simulink library "monroe_library"  (R2012b)
settings: Solver=ode45  StartTime=0.0  StopTime=10.0  RelTol=1e-3
values from neighbouring files (symbols this model uses):
  input_bit_width = ', num2str(input_bit_width))    [fft_direct_draw.m]
undefined symbols (not defined in the file or in its folder): gcbh, xlBlockLoadCallback
libraries: xbsIndex_r4 x1880, monroe_library x159, casper_library x13, xps_library x1
(part 35 of 43)

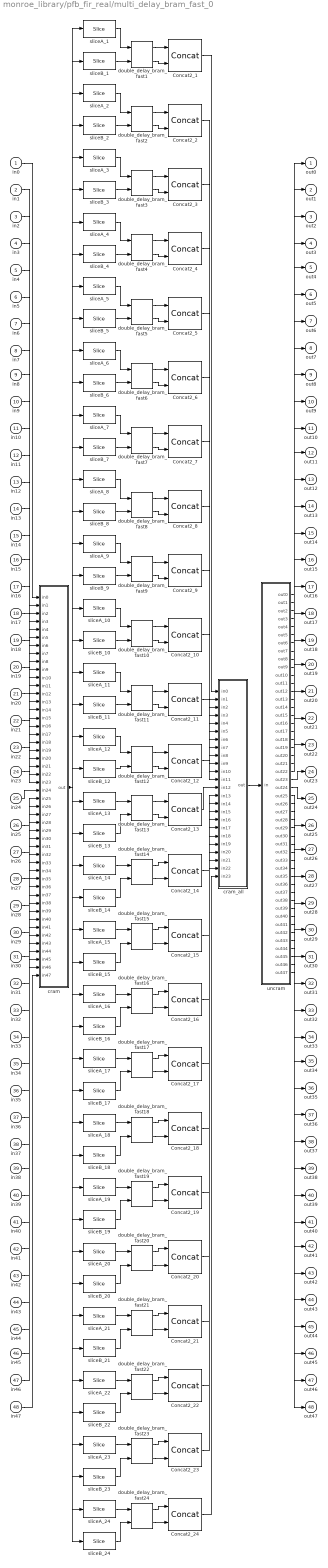
== system monroe_library/pfb_fir_real/multi_delay_bram_fast_0 ==
  in0 : Inport
  in1 : Inport  Port=2
  in2 : Inport  Port=3
  in3 : Inport  Port=4
  in4 : Inport  Port=5
  in5 : Inport  Port=6
  in6 : Inport  Port=7
  in7 : Inport  Port=8
  in8 : Inport  Port=9
  in9 : Inport  Port=10
  in10 : Inport  Port=11
  in11 : Inport  Port=12
  in12 : Inport  Port=13
  in13 : Inport  Port=14
  in14 : Inport  Port=15
  in15 : Inport  Port=16
  in16 : Inport  Port=17
  in17 : Inport  Port=18
  in18 : Inport  Port=19
  in19 : Inport  Port=20
  in20 : Inport  Port=21
  in21 : Inport  Port=22
  in22 : Inport  Port=23
  in23 : Inport  Port=24
  in24 : Inport  Port=25
  in25 : Inport  Port=26
  in26 : Inport  Port=27
  in27 : Inport  Port=28
  in28 : Inport  Port=29
  in29 : Inport  Port=30
  in30 : Inport  Port=31
  in31 : Inport  Port=32
  in32 : Inport  Port=33
  in33 : Inport  Port=34
  in34 : Inport  Port=35
  in35 : Inport  Port=36
  in36 : Inport  Port=37
  in37 : Inport  Port=38
  in38 : Inport  Port=39
  in39 : Inport  Port=40
  in40 : Inport  Port=41
  in41 : Inport  Port=42
  in42 : Inport  Port=43
  in43 : Inport  Port=44
  in44 : Inport  Port=45
  in45 : Inport  Port=46
  in46 : Inport  Port=47
  in47 : Inport  Port=48
  Concat2_{1..24} (24 alike) : xbsIndex_r4/Concat  num_inputs=2  dbl_ovrd=off  block_type=concat
  cram : Subsystem
  cram_all : Subsystem
  double_delay_bram_fast{1..24} (24 alike) : monroe_library/double_delay_bram_fast  SystemSampleTime=-1  delay_len=1024  bram_latency=2  register_counter=0
  sliceA_1 : xbsIndex_r4/Slice  nbits=18  boolean_output=off  mode=Upper Bit Location + Width  bit1=-0  base1=MSB of Input  bit0=-0  base0=MSB of Input  dbl_ovrd=off  block_type=slice
  sliceA_10 : xbsIndex_r4/Slice  nbits=18  boolean_output=off  mode=Upper Bit Location + Width  bit1=-324  base1=MSB of Input  bit0=-324  base0=MSB of Input  dbl_ovrd=off  block_type=slice
  sliceA_11 : xbsIndex_r4/Slice  nbits=18  boolean_output=off  mode=Upper Bit Location + Width  bit1=-360  base1=MSB of Input  bit0=-360  base0=MSB of Input  dbl_ovrd=off  block_type=slice
  sliceA_12 : xbsIndex_r4/Slice  nbits=18  boolean_output=off  mode=Upper Bit Location + Width  bit1=-396  base1=MSB of Input  bit0=-396  base0=MSB of Input  dbl_ovrd=off  block_type=slice
  sliceA_13 : xbsIndex_r4/Slice  nbits=18  boolean_output=off  mode=Upper Bit Location + Width  bit1=-432  base1=MSB of Input  bit0=-432  base0=MSB of Input  dbl_ovrd=off  block_type=slice
  sliceA_14 : xbsIndex_r4/Slice  nbits=18  boolean_output=off  mode=Upper Bit Location + Width  bit1=-468  base1=MSB of Input  bit0=-468  base0=MSB of Input  dbl_ovrd=off  block_type=slice
  sliceA_15 : xbsIndex_r4/Slice  nbits=18  boolean_output=off  mode=Upper Bit Location + Width  bit1=-504  base1=MSB of Input  bit0=-504  base0=MSB of Input  dbl_ovrd=off  block_type=slice
  sliceA_16 : xbsIndex_r4/Slice  nbits=18  boolean_output=off  mode=Upper Bit Location + Width  bit1=-540  base1=MSB of Input  bit0=-540  base0=MSB of Input  dbl_ovrd=off  block_type=slice
  sliceA_17 : xbsIndex_r4/Slice  nbits=18  boolean_output=off  mode=Upper Bit Location + Width  bit1=-576  base1=MSB of Input  bit0=-576  base0=MSB of Input  dbl_ovrd=off  block_type=slice
  sliceA_18 : xbsIndex_r4/Slice  nbits=18  boolean_output=off  mode=Upper Bit Location + Width  bit1=-612  base1=MSB of Input  bit0=-612  base0=MSB of Input  dbl_ovrd=off  block_type=slice
  sliceA_19 : xbsIndex_r4/Slice  nbits=18  boolean_output=off  mode=Upper Bit Location + Width  bit1=-648  base1=MSB of Input  bit0=-648  base0=MSB of Input  dbl_ovrd=off  block_type=slice
  sliceA_2 : xbsIndex_r4/Slice  nbits=18  boolean_output=off  mode=Upper Bit Location + Width  bit1=-36  base1=MSB of Input  bit0=-36  base0=MSB of Input  dbl_ovrd=off  block_type=slice
  sliceA_20 : xbsIndex_r4/Slice  nbits=18  boolean_output=off  mode=Upper Bit Location + Width  bit1=-684  base1=MSB of Input  bit0=-684  base0=MSB of Input  dbl_ovrd=off  block_type=slice
  sliceA_21 : xbsIndex_r4/Slice  nbits=18  boolean_output=off  mode=Upper Bit Location + Width  bit1=-720  base1=MSB of Input  bit0=-720  base0=MSB of Input  dbl_ovrd=off  block_type=slice
  sliceA_22 : xbsIndex_r4/Slice  nbits=18  boolean_output=off  mode=Upper Bit Location + Width  bit1=-756  base1=MSB of Input  bit0=-756  base0=MSB of Input  dbl_ovrd=off  block_type=slice
  sliceA_23 : xbsIndex_r4/Slice  nbits=18  boolean_output=off  mode=Upper Bit Location + Width  bit1=-792  base1=MSB of Input  bit0=-792  base0=MSB of Input  dbl_ovrd=off  block_type=slice
  sliceA_24 : xbsIndex_r4/Slice  nbits=18  boolean_output=off  mode=Upper Bit Location + Width  bit1=-828  base1=MSB of Input  bit0=-828  base0=MSB of Input  dbl_ovrd=off  block_type=slice
  sliceA_3 : xbsIndex_r4/Slice  nbits=18  boolean_output=off  mode=Upper Bit Location + Width  bit1=-72  base1=MSB of Input  bit0=-72  base0=MSB of Input  dbl_ovrd=off  block_type=slice
  sliceA_4 : xbsIndex_r4/Slice  nbits=18  boolean_output=off  mode=Upper Bit Location + Width  bit1=-108  base1=MSB of Input  bit0=-108  base0=MSB of Input  dbl_ovrd=off  block_type=slice
  sliceA_5 : xbsIndex_r4/Slice  nbits=18  boolean_output=off  mode=Upper Bit Location + Width  bit1=-144  base1=MSB of Input  bit0=-144  base0=MSB of Input  dbl_ovrd=off  block_type=slice
  sliceA_6 : xbsIndex_r4/Slice  nbits=18  boolean_output=off  mode=Upper Bit Location + Width  bit1=-180  base1=MSB of Input  bit0=-180  base0=MSB of Input  dbl_ovrd=off  block_type=slice
  sliceA_7 : xbsIndex_r4/Slice  nbits=18  boolean_output=off  mode=Upper Bit Location + Width  bit1=-216  base1=MSB of Input  bit0=-216  base0=MSB of Input  dbl_ovrd=off  block_type=slice
  sliceA_8 : xbsIndex_r4/Slice  nbits=18  boolean_output=off  mode=Upper Bit Location + Width  bit1=-252  base1=MSB of Input  bit0=-252  base0=MSB of Input  dbl_ovrd=off  block_type=slice
  sliceA_9 : xbsIndex_r4/Slice  nbits=18  boolean_output=off  mode=Upper Bit Location + Width  bit1=-288  base1=MSB of Input  bit0=-288  base0=MSB of Input  dbl_ovrd=off  block_type=slice
  sliceB_1 : xbsIndex_r4/Slice  nbits=18  boolean_output=off  mode=Upper Bit Location + Width  bit1=-18  base1=MSB of Input  bit0=-18  base0=MSB of Input  dbl_ovrd=off  block_type=slice
  sliceB_10 : xbsIndex_r4/Slice  nbits=18  boolean_output=off  mode=Upper Bit Location + Width  bit1=-342  base1=MSB of Input  bit0=-342  base0=MSB of Input  dbl_ovrd=off  block_type=slice
  sliceB_11 : xbsIndex_r4/Slice  nbits=18  boolean_output=off  mode=Upper Bit Location + Width  bit1=-378  base1=MSB of Input  bit0=-378  base0=MSB of Input  dbl_ovrd=off  block_type=slice
  sliceB_12 : xbsIndex_r4/Slice  nbits=18  boolean_output=off  mode=Upper Bit Location + Width  bit1=-414  base1=MSB of Input  bit0=-414  base0=MSB of Input  dbl_ovrd=off  block_type=slice
  sliceB_13 : xbsIndex_r4/Slice  nbits=18  boolean_output=off  mode=Upper Bit Location + Width  bit1=-450  base1=MSB of Input  bit0=-450  base0=MSB of Input  dbl_ovrd=off  block_type=slice
  sliceB_14 : xbsIndex_r4/Slice  nbits=18  boolean_output=off  mode=Upper Bit Location + Width  bit1=-486  base1=MSB of Input  bit0=-486  base0=MSB of Input  dbl_ovrd=off  block_type=slice
  sliceB_15 : xbsIndex_r4/Slice  nbits=18  boolean_output=off  mode=Upper Bit Location + Width  bit1=-522  base1=MSB of Input  bit0=-522  base0=MSB of Input  dbl_ovrd=off  block_type=slice
  sliceB_16 : xbsIndex_r4/Slice  nbits=18  boolean_output=off  mode=Upper Bit Location + Width  bit1=-558  base1=MSB of Input  bit0=-558  base0=MSB of Input  dbl_ovrd=off  block_type=slice
  sliceB_17 : xbsIndex_r4/Slice  nbits=18  boolean_output=off  mode=Upper Bit Location + Width  bit1=-594  base1=MSB of Input  bit0=-594  base0=MSB of Input  dbl_ovrd=off  block_type=slice
  sliceB_18 : xbsIndex_r4/Slice  nbits=18  boolean_output=off  mode=Upper Bit Location + Width  bit1=-630  base1=MSB of Input  bit0=-630  base0=MSB of Input  dbl_ovrd=off  block_type=slice
  sliceB_19 : xbsIndex_r4/Slice  nbits=18  boolean_output=off  mode=Upper Bit Location + Width  bit1=-666  base1=MSB of Input  bit0=-666  base0=MSB of Input  dbl_ovrd=off  block_type=slice
  sliceB_2 : xbsIndex_r4/Slice  nbits=18  boolean_output=off  mode=Upper Bit Location + Width  bit1=-54  base1=MSB of Input  bit0=-54  base0=MSB of Input  dbl_ovrd=off  block_type=slice
  sliceB_20 : xbsIndex_r4/Slice  nbits=18  boolean_output=off  mode=Upper Bit Location + Width  bit1=-702  base1=MSB of Input  bit0=-702  base0=MSB of Input  dbl_ovrd=off  block_type=slice
  sliceB_21 : xbsIndex_r4/Slice  nbits=18  boolean_output=off  mode=Upper Bit Location + Width  bit1=-738  base1=MSB of Input  bit0=-738  base0=MSB of Input  dbl_ovrd=off  block_type=slice
  sliceB_22 : xbsIndex_r4/Slice  nbits=18  boolean_output=off  mode=Upper Bit Location + Width  bit1=-774  base1=MSB of Input  bit0=-774  base0=MSB of Input  dbl_ovrd=off  block_type=slice
  sliceB_23 : xbsIndex_r4/Slice  nbits=18  boolean_output=off  mode=Upper Bit Location + Width  bit1=-810  base1=MSB of Input  bit0=-810  base0=MSB of Input  dbl_ovrd=off  block_type=slice
  sliceB_24 : xbsIndex_r4/Slice  nbits=18  boolean_output=off  mode=Upper Bit Location + Width  bit1=-846  base1=MSB of Input  bit0=-846  base0=MSB of Input  dbl_ovrd=off  block_type=slice
  sliceB_3 : xbsIndex_r4/Slice  nbits=18  boolean_output=off  mode=Upper Bit Location + Width  bit1=-90  base1=MSB of Input  bit0=-90  base0=MSB of Input  dbl_ovrd=off  block_type=slice
  sliceB_4 : xbsIndex_r4/Slice  nbits=18  boolean_output=off  mode=Upper Bit Location + Width  bit1=-126  base1=MSB of Input  bit0=-126  base0=MSB of Input  dbl_ovrd=off  block_type=slice
  sliceB_5 : xbsIndex_r4/Slice  nbits=18  boolean_output=off  mode=Upper Bit Location + Width  bit1=-162  base1=MSB of Input  bit0=-162  base0=MSB of Input  dbl_ovrd=off  block_type=slice
  sliceB_6 : xbsIndex_r4/Slice  nbits=18  boolean_output=off  mode=Upper Bit Location + Width  bit1=-198  base1=MSB of Input  bit0=-198  base0=MSB of Input  dbl_ovrd=off  block_type=slice
  sliceB_7 : xbsIndex_r4/Slice  nbits=18  boolean_output=off  mode=Upper Bit Location + Width  bit1=-234  base1=MSB of Input  bit0=-234  base0=MSB of Input  dbl_ovrd=off  block_type=slice
  sliceB_8 : xbsIndex_r4/Slice  nbits=18  boolean_output=off  mode=Upper Bit Location + Width  bit1=-270  base1=MSB of Input  bit0=-270  base0=MSB of Input  dbl_ovrd=off  block_type=slice
  sliceB_9 : xbsIndex_r4/Slice  nbits=18  boolean_output=off  mode=Upper Bit Location + Width  bit1=-306  base1=MSB of Input  bit0=-306  base0=MSB of Input  dbl_ovrd=off  block_type=slice
  uncram : Subsystem
  out0 : Outport
  out1 : Outport  Port=2
  out2 : Outport  Port=3
  out3 : Outport  Port=4
  out4 : Outport  Port=5
  out5 : Outport  Port=6
  out6 : Outport  Port=7
  out7 : Outport  Port=8
  out8 : Outport  Port=9
  out9 : Outport  Port=10
  out10 : Outport  Port=11
  out11 : Outport  Port=12
  out12 : Outport  Port=13
  out13 : Outport  Port=14
  out14 : Outport  Port=15
  out15 : Outport  Port=16
  out16 : Outport  Port=17
  out17 : Outport  Port=18
  out18 : Outport  Port=19
  out19 : Outport  Port=20
  out20 : Outport  Port=21
  out21 : Outport  Port=22
  out22 : Outport  Port=23
  out23 : Outport  Port=24
  out24 : Outport  Port=25
  out25 : Outport  Port=26
  out26 : Outport  Port=27
  out27 : Outport  Port=28
  out28 : Outport  Port=29
  out29 : Outport  Port=30
  out30 : Outport  Port=31
  out31 : Outport  Port=32
  out32 : Outport  Port=33
  out33 : Outport  Port=34
  out34 : Outport  Port=35
  out35 : Outport  Port=36
  out36 : Outport  Port=37
  out37 : Outport  Port=38
  out38 : Outport  Port=39
  out39 : Outport  Port=40
  out40 : Outport  Port=41
  out41 : Outport  Port=42
  out42 : Outport  Port=43
  out43 : Outport  Port=44
  out44 : Outport  Port=45
  out45 : Outport  Port=46
  out46 : Outport  Port=47
  out47 : Outport  Port=48
  wires:
  cram/1(out) -> sliceB_24/1, sliceA_24/1, sliceB_23/1, sliceA_23/1, sliceB_22/1, sliceA_22/1, sliceB_21/1, sliceA_21/1, sliceB_20/1, sliceA_20/1, sliceB_19/1, sliceA_19/1, sliceB_18/1, sliceA_18/1, sliceB_17/1, sliceA_17/1, sliceB_16/1, sliceA_16/1, sliceB_15/1, sliceA_15/1, sliceB_14/1, sliceA_14/1, sliceB_13/1, sliceA_13/1, sliceB_12/1, sliceA_12/1, sliceB_11/1, sliceA_11/1, sliceB_10/1, sliceA_10/1, sliceB_9/1, sliceA_9/1, sliceB_8/1, sliceA_8/1, sliceB_7/1, sliceA_7/1, sliceB_6/1, sliceA_6/1, sliceB_5/1, sliceA_5/1, sliceB_4/1, sliceA_4/1, sliceB_3/1, sliceA_3/1, sliceB_2/1, sliceA_2/1, sliceB_1/1, sliceA_1/1
  uncram/48(out47) -> out47/1
  uncram/47(out46) -> out46/1
  uncram/46(out45) -> out45/1
  uncram/45(out44) -> out44/1
  uncram/44(out43) -> out43/1
  uncram/43(out42) -> out42/1
  uncram/42(out41) -> out41/1
  uncram/41(out40) -> out40/1
  uncram/40(out39) -> out39/1
  uncram/39(out38) -> out38/1
  uncram/38(out37) -> out37/1
  uncram/37(out36) -> out36/1
  uncram/36(out35) -> out35/1
  uncram/35(out34) -> out34/1
  uncram/34(out33) -> out33/1
  uncram/33(out32) -> out32/1
  uncram/32(out31) -> out31/1
  uncram/31(out30) -> out30/1
  uncram/30(out29) -> out29/1
  uncram/29(out28) -> out28/1
  uncram/28(out27) -> out27/1
  uncram/27(out26) -> out26/1
  uncram/26(out25) -> out25/1
  uncram/25(out24) -> out24/1
  uncram/24(out23) -> out23/1
  uncram/23(out22) -> out22/1
  uncram/22(out21) -> out21/1
  uncram/21(out20) -> out20/1
  uncram/20(out19) -> out19/1
  uncram/19(out18) -> out18/1
  uncram/18(out17) -> out17/1
  uncram/17(out16) -> out16/1
  uncram/16(out15) -> out15/1
  uncram/15(out14) -> out14/1
  uncram/14(out13) -> out13/1
  uncram/13(out12) -> out12/1
  uncram/12(out11) -> out11/1
  uncram/11(out10) -> out10/1
  uncram/10(out9) -> out9/1
  uncram/9(out8) -> out8/1
  uncram/8(out7) -> out7/1
  uncram/7(out6) -> out6/1
  uncram/6(out5) -> out5/1
  uncram/5(out4) -> out4/1
  uncram/4(out3) -> out3/1
  uncram/3(out2) -> out2/1
  uncram/2(out1) -> out1/1
  uncram/1(out0) -> out0/1
  cram_all/1(out) -> uncram/1(in)
  Concat2_24/1 -> cram_all/24(in23)
  Concat2_23/1 -> cram_all/23(in22)
  Concat2_22/1 -> cram_all/22(in21)
  Concat2_21/1 -> cram_all/21(in20)
  Concat2_20/1 -> cram_all/20(in19)
  Concat2_19/1 -> cram_all/19(in18)
  Concat2_18/1 -> cram_all/18(in17)
  Concat2_17/1 -> cram_all/17(in16)
  Concat2_16/1 -> cram_all/16(in15)
  Concat2_15/1 -> cram_all/15(in14)
  Concat2_14/1 -> cram_all/14(in13)
  Concat2_13/1 -> cram_all/13(in12)
  Concat2_12/1 -> cram_all/12(in11)
  Concat2_11/1 -> cram_all/11(in10)
  Concat2_10/1 -> cram_all/10(in9)
  Concat2_9/1 -> cram_all/9(in8)
  Concat2_8/1 -> cram_all/8(in7)
  Concat2_7/1 -> cram_all/7(in6)
  Concat2_6/1 -> cram_all/6(in5)
  Concat2_5/1 -> cram_all/5(in4)
  Concat2_4/1 -> cram_all/4(in3)
  Concat2_3/1 -> cram_all/3(in2)
  Concat2_2/1 -> cram_all/2(in1)
  Concat2_1/1 -> cram_all/1(in0)
  double_delay_bram_fast24/2 -> Concat2_24/2
  double_delay_bram_fast24/1 -> Concat2_24/1
  sliceB_24/1 -> double_delay_bram_fast24/2
  sliceA_24/1 -> double_delay_bram_fast24/1
  double_delay_bram_fast23/2 -> Concat2_23/2
  double_delay_bram_fast23/1 -> Concat2_23/1
  sliceB_23/1 -> double_delay_bram_fast23/2
  sliceA_23/1 -> double_delay_bram_fast23/1
  double_delay_bram_fast22/2 -> Concat2_22/2
  double_delay_bram_fast22/1 -> Concat2_22/1
  sliceB_22/1 -> double_delay_bram_fast22/2
  sliceA_22/1 -> double_delay_bram_fast22/1
  double_delay_bram_fast21/2 -> Concat2_21/2
  double_delay_bram_fast21/1 -> Concat2_21/1
  sliceB_21/1 -> double_delay_bram_fast21/2
  sliceA_21/1 -> double_delay_bram_fast21/1
  double_delay_bram_fast20/2 -> Concat2_20/2
  double_delay_bram_fast20/1 -> Concat2_20/1
  sliceB_20/1 -> double_delay_bram_fast20/2
  sliceA_20/1 -> double_delay_bram_fast20/1
  double_delay_bram_fast19/2 -> Concat2_19/2
  double_delay_bram_fast19/1 -> Concat2_19/1
  sliceB_19/1 -> double_delay_bram_fast19/2
  sliceA_19/1 -> double_delay_bram_fast19/1
  double_delay_bram_fast18/2 -> Concat2_18/2
  double_delay_bram_fast18/1 -> Concat2_18/1
  sliceB_18/1 -> double_delay_bram_fast18/2
  sliceA_18/1 -> double_delay_bram_fast18/1
  double_delay_bram_fast17/2 -> Concat2_17/2
  double_delay_bram_fast17/1 -> Concat2_17/1
  sliceB_17/1 -> double_delay_bram_fast17/2
  sliceA_17/1 -> double_delay_bram_fast17/1
  double_delay_bram_fast16/2 -> Concat2_16/2
  double_delay_bram_fast16/1 -> Concat2_16/1
  sliceB_16/1 -> double_delay_bram_fast16/2
  sliceA_16/1 -> double_delay_bram_fast16/1
  double_delay_bram_fast15/2 -> Concat2_15/2
  double_delay_bram_fast15/1 -> Concat2_15/1
  sliceB_15/1 -> double_delay_bram_fast15/2
  sliceA_15/1 -> double_delay_bram_fast15/1
  double_delay_bram_fast14/2 -> Concat2_14/2
  double_delay_bram_fast14/1 -> Concat2_14/1
  sliceB_14/1 -> double_delay_bram_fast14/2
  sliceA_14/1 -> double_delay_bram_fast14/1
  double_delay_bram_fast13/2 -> Concat2_13/2
  double_delay_bram_fast13/1 -> Concat2_13/1
  sliceB_13/1 -> double_delay_bram_fast13/2
  sliceA_13/1 -> double_delay_bram_fast13/1
  double_delay_bram_fast12/2 -> Concat2_12/2
  double_delay_bram_fast12/1 -> Concat2_12/1
  sliceB_12/1 -> double_delay_bram_fast12/2
  sliceA_12/1 -> double_delay_bram_fast12/1
  double_delay_bram_fast11/2 -> Concat2_11/2
  double_delay_bram_fast11/1 -> Concat2_11/1
  sliceB_11/1 -> double_delay_bram_fast11/2
  sliceA_11/1 -> double_delay_bram_fast11/1
  double_delay_bram_fast10/2 -> Concat2_10/2
  double_delay_bram_fast10/1 -> Concat2_10/1
  sliceB_10/1 -> double_delay_bram_fast10/2
  sliceA_10/1 -> double_delay_bram_fast10/1
  double_delay_bram_fast9/2 -> Concat2_9/2
  double_delay_bram_fast9/1 -> Concat2_9/1
  sliceB_9/1 -> double_delay_bram_fast9/2
  sliceA_9/1 -> double_delay_bram_fast9/1
  double_delay_bram_fast8/2 -> Concat2_8/2
  double_delay_bram_fast8/1 -> Concat2_8/1
  sliceB_8/1 -> double_delay_bram_fast8/2
  sliceA_8/1 -> double_delay_bram_fast8/1
  double_delay_bram_fast7/2 -> Concat2_7/2
  double_delay_bram_fast7/1 -> Concat2_7/1
  sliceB_7/1 -> double_delay_bram_fast7/2
  sliceA_7/1 -> double_delay_bram_fast7/1
  double_delay_bram_fast6/2 -> Concat2_6/2
  double_delay_bram_fast6/1 -> Concat2_6/1
  sliceB_6/1 -> double_delay_bram_fast6/2
  sliceA_6/1 -> double_delay_bram_fast6/1
  double_delay_bram_fast5/2 -> Concat2_5/2
  double_delay_bram_fast5/1 -> Concat2_5/1
  sliceB_5/1 -> double_delay_bram_fast5/2
  sliceA_5/1 -> double_delay_bram_fast5/1
  double_delay_bram_fast4/2 -> Concat2_4/2
  double_delay_bram_fast4/1 -> Concat2_4/1
  sliceB_4/1 -> double_delay_bram_fast4/2
  sliceA_4/1 -> double_delay_bram_fast4/1
  double_delay_bram_fast3/2 -> Concat2_3/2
  double_delay_bram_fast3/1 -> Concat2_3/1
  sliceB_3/1 -> double_delay_bram_fast3/2
  sliceA_3/1 -> double_delay_bram_fast3/1
  double_delay_bram_fast2/2 -> Concat2_2/2
  double_delay_bram_fast2/1 -> Concat2_2/1
  sliceB_2/1 -> double_delay_bram_fast2/2
  sliceA_2/1 -> double_delay_bram_fast2/1
  double_delay_bram_fast1/2 -> Concat2_1/2
  double_delay_bram_fast1/1 -> Concat2_1/1
  sliceB_1/1 -> double_delay_bram_fast1/2
  sliceA_1/1 -> double_delay_bram_fast1/1
  in47/1 -> cram/48(in47)
  in46/1 -> cram/47(in46)
  in45/1 -> cram/46(in45)
  in44/1 -> cram/45(in44)
  in43/1 -> cram/44(in43)
  in42/1 -> cram/43(in42)
  in41/1 -> cram/42(in41)
  in40/1 -> cram/41(in40)
  in39/1 -> cram/40(in39)
  in38/1 -> cram/39(in38)
  in37/1 -> cram/38(in37)
  in36/1 -> cram/37(in36)
  in35/1 -> cram/36(in35)
  in34/1 -> cram/35(in34)
  in33/1 -> cram/34(in33)
  in32/1 -> cram/33(in32)
  in31/1 -> cram/32(in31)
  in30/1 -> cram/31(in30)
  in29/1 -> cram/30(in29)
  in28/1 -> cram/29(in28)
  in27/1 -> cram/28(in27)
  in26/1 -> cram/27(in26)
  in25/1 -> cram/26(in25)
  in24/1 -> cram/25(in24)
  in23/1 -> cram/24(in23)
  in22/1 -> cram/23(in22)
  in21/1 -> cram/22(in21)
  in20/1 -> cram/21(in20)
  in19/1 -> cram/20(in19)
  in18/1 -> cram/19(in18)
  in17/1 -> cram/18(in17)
  in16/1 -> cram/17(in16)
  in15/1 -> cram/16(in15)
  in14/1 -> cram/15(in14)
  in13/1 -> cram/14(in13)
  in12/1 -> cram/13(in12)
  in11/1 -> cram/12(in11)
  in10/1 -> cram/11(in10)
  in9/1 -> cram/10(in9)
  in8/1 -> cram/9(in8)
  in7/1 -> cram/8(in7)
  in6/1 -> cram/7(in6)
  in5/1 -> cram/6(in5)
  in4/1 -> cram/5(in4)
  in3/1 -> cram/4(in3)
  in2/1 -> cram/3(in2)
  in1/1 -> cram/2(in1)
  in0/1 -> cram/1(in0)

== system monroe_library/twiddle_cheap/c_to_ri1 ==
  c : Inport
  force_im : xbsIndex_r4/Reinterpret  force_arith_type=on  arith_type="Signed  (2's comp)"  force_bin_pt=on  bin_pt=bin_pt  block_type=reinterpret
      settings: infoedit="Changes signal type without altering the binary representation.   You can changed the signal between signed and unsigned, and relocate the binary point.<P><P>Hardware notes: In hardware this block costs nothing.<P><P>Example:  Suppose the input is 6 bits wide, signed, with 2 fractional bits, and the output is forced to unsigned with 0 fractional bits.  Then an input of -2.0 (1110.00 in binary 2's complement) becomes an output of 56 (111000 in binary)."  block_version=9.1.01
  force_re : xbsIndex_r4/Reinterpret  force_arith_type=on  arith_type="Signed  (2's comp)"  force_bin_pt=on  bin_pt=bin_pt  block_type=reinterpret
      settings: infoedit="Changes signal type without altering the binary representation.   You can changed the signal between signed and unsigned, and relocate the binary point.<P><P>Hardware notes: In hardware this block costs nothing.<P><P>Example:  Suppose the input is 6 bits wide, signed, with 2 fractional bits, and the output is forced to unsigned with 0 fractional bits.  Then an input of -2.0 (1110.00 in binary 2's complement) becomes an output of 56 (111000 in binary)."  block_version=9.1.01
  slice_im : xbsIndex_r4/Slice  nbits=n_bits  boolean_output=off  mode=Lower Bit Location + Width  bit1=0  base1=MSB of Input  bit0=0  base0=LSB of Input  dbl_ovrd=off  block_type=slice
      settings: infoedit="Extracts a given range of bits from each input sample and presents it at the output.  The output type is ordinarily unsigned with binary point at zero, but can be Boolean when the slice is one bit wide.<P><P>Hardware notes: In hardware this block costs nothing."  block_version=9.1.01
  slice_re : xbsIndex_r4/Slice  nbits=n_bits  boolean_output=off  mode=Upper Bit Location + Width  bit1=0  base1=MSB of Input  bit0=0  base0=LSB of Input  dbl_ovrd=off  block_type=slice
      settings: infoedit="Extracts a given range of bits from each input sample and presents it at the output.  The output type is ordinarily unsigned with binary point at zero, but can be Boolean when the slice is one bit wide.<P><P>Hardware notes: In hardware this block costs nothing."  block_version=9.1.01
  re : Outport
  im : Outport  Port=2
  wires:
  c/1 -> slice_im/1, slice_re/1
  force_im/1 -> im/1
  force_re/1 -> re/1
  slice_im/1 -> force_im/1
  slice_re/1 -> force_re/1

== system monroe_library/twiddle_cheap/c_to_ri2 ==
  c : Inport
  force_im : xbsIndex_r4/Reinterpret  force_arith_type=on  arith_type="Signed  (2's comp)"  force_bin_pt=on  bin_pt=bin_pt  block_type=reinterpret
      settings: infoedit="Changes signal type without altering the binary representation.   You can changed the signal between signed and unsigned, and relocate the binary point.<P><P>Hardware notes: In hardware this block costs nothing.<P><P>Example:  Suppose the input is 6 bits wide, signed, with 2 fractional bits, and the output is forced to unsigned with 0 fractional bits.  Then an input of -2.0 (1110.00 in binary 2's complement) becomes an output of 56 (111000 in binary)."  block_version=9.1.01
  force_re : xbsIndex_r4/Reinterpret  force_arith_type=on  arith_type="Signed  (2's comp)"  force_bin_pt=on  bin_pt=bin_pt  block_type=reinterpret
      settings: infoedit="Changes signal type without altering the binary representation.   You can changed the signal between signed and unsigned, and relocate the binary point.<P><P>Hardware notes: In hardware this block costs nothing.<P><P>Example:  Suppose the input is 6 bits wide, signed, with 2 fractional bits, and the output is forced to unsigned with 0 fractional bits.  Then an input of -2.0 (1110.00 in binary 2's complement) becomes an output of 56 (111000 in binary)."  block_version=9.1.01
  slice_im : xbsIndex_r4/Slice  nbits=n_bits  boolean_output=off  mode=Lower Bit Location + Width  bit1=0  base1=MSB of Input  bit0=0  base0=LSB of Input  dbl_ovrd=off  block_type=slice
      settings: infoedit="Extracts a given range of bits from each input sample and presents it at the output.  The output type is ordinarily unsigned with binary point at zero, but can be Boolean when the slice is one bit wide.<P><P>Hardware notes: In hardware this block costs nothing."  block_version=9.1.01
  slice_re : xbsIndex_r4/Slice  nbits=n_bits  boolean_output=off  mode=Upper Bit Location + Width  bit1=0  base1=MSB of Input  bit0=0  base0=LSB of Input  dbl_ovrd=off  block_type=slice
      settings: infoedit="Extracts a given range of bits from each input sample and presents it at the output.  The output type is ordinarily unsigned with binary point at zero, but can be Boolean when the slice is one bit wide.<P><P>Hardware notes: In hardware this block costs nothing."  block_version=9.1.01
  re : Outport
  im : Outport  Port=2
  wires:
  slice_re/1 -> force_re/1
  slice_im/1 -> force_im/1
  force_re/1 -> re/1
  force_im/1 -> im/1
  c/1 -> slice_re/1, slice_im/1

== system monroe_library/twiddle_cheap/c_to_ri3 ==
  c : Inport
  force_im : xbsIndex_r4/Reinterpret  force_arith_type=on  arith_type="Signed  (2's comp)"  force_bin_pt=on  bin_pt=bin_pt  block_type=reinterpret
      settings: infoedit="Changes signal type without altering the binary representation.   You can changed the signal between signed and unsigned, and relocate the binary point.<P><P>Hardware notes: In hardware this block costs nothing.<P><P>Example:  Suppose the input is 6 bits wide, signed, with 2 fractional bits, and the output is forced to unsigned with 0 fractional bits.  Then an input of -2.0 (1110.00 in binary 2's complement) becomes an output of 56 (111000 in binary)."  block_version=9.1.01
  force_re : xbsIndex_r4/Reinterpret  force_arith_type=on  arith_type="Signed  (2's comp)"  force_bin_pt=on  bin_pt=bin_pt  block_type=reinterpret
      settings: infoedit="Changes signal type without altering the binary representation.   You can changed the signal between signed and unsigned, and relocate the binary point.<P><P>Hardware notes: In hardware this block costs nothing.<P><P>Example:  Suppose the input is 6 bits wide, signed, with 2 fractional bits, and the output is forced to unsigned with 0 fractional bits.  Then an input of -2.0 (1110.00 in binary 2's complement) becomes an output of 56 (111000 in binary)."  block_version=9.1.01
  slice_im : xbsIndex_r4/Slice  nbits=n_bits  boolean_output=off  mode=Lower Bit Location + Width  bit1=0  base1=MSB of Input  bit0=0  base0=LSB of Input  dbl_ovrd=off  block_type=slice
      settings: infoedit="Extracts a given range of bits from each input sample and presents it at the output.  The output type is ordinarily unsigned with binary point at zero, but can be Boolean when the slice is one bit wide.<P><P>Hardware notes: In hardware this block costs nothing."  block_version=9.1.01
  slice_re : xbsIndex_r4/Slice  nbits=n_bits  boolean_output=off  mode=Upper Bit Location + Width  bit1=0  base1=MSB of Input  bit0=0  base0=LSB of Input  dbl_ovrd=off  block_type=slice
      settings: infoedit="Extracts a given range of bits from each input sample and presents it at the output.  The output type is ordinarily unsigned with binary point at zero, but can be Boolean when the slice is one bit wide.<P><P>Hardware notes: In hardware this block costs nothing."  block_version=9.1.01
  re : Outport
  im : Outport  Port=2
  wires:
  c/1 -> slice_im/1, slice_re/1
  force_im/1 -> im/1
  force_re/1 -> re/1
  slice_im/1 -> force_im/1
  slice_re/1 -> force_re/1

== system monroe_library/twiddle_stage2/negate_dsp48 ==
  In1 : Inport
  Convert : xbsIndex_r4/Convert  arith_type="Signed  (2's comp)"  n_bits=30  bin_pt=input_bin_pt  quantization=Truncate  overflow=Wrap  en=off  latency=0  dbl_ovrd=off  pipeline=off  block_type=convert
      settings: block_version=11.4
  Convert1 : xbsIndex_r4/Convert  arith_type="Signed  (2's comp)"  n_bits=input_bit_width  bin_pt=input_bin_pt  quantization=Truncate  overflow=Wrap  en=off  latency=0  dbl_ovrd=off  pipeline=off  block_type=convert
      settings: block_version=11.4
  Reinterpret : xbsIndex_r4/Reinterpret  force_arith_type=on  arith_type="Signed  (2's comp)"  force_bin_pt=on  bin_pt=input_bin_pt  block_type=reinterpret
      settings: infoedit="Changes signal type without altering the binary representation.   You can changed the signal between signed and unsigned, and relocate the binary point.<br><br>Hardware notes: In hardware this block costs nothing.<br><br>Example:  Suppose the input is 6 bits wide, signed, with 2 fractional bits, and the output is forced to unsigned with 0 fractional bits.  Then an input of -2.0 (1110.00 in binary 2's complement) becomes an output of 56 (111000 in binary)."
  Reinterpret1 : xbsIndex_r4/Reinterpret  force_arith_type=on  arith_type="Signed  (2's comp)"  force_bin_pt=on  bin_pt=0  block_type=reinterpret
      settings: infoedit="Changes signal type without altering the binary representation.   You can changed the signal between signed and unsigned, and relocate the binary point.<br><br>Hardware notes: In hardware this block costs nothing.<br><br>Example:  Suppose the input is 6 bits wide, signed, with 2 fractional bits, and the output is forced to unsigned with 0 fractional bits.  Then an input of -2.0 (1110.00 in binary 2's complement) becomes an output of 56 (111000 in binary)."
  alucode3 : xbsIndex_r4/Constant  arith_type=Unsigned  const=0  n_bits=4  bin_pt=0  explicit_period=on  period=1  equ=P=C  opselect=C  inp2=PCIN>>17  opr=+  inp1=P  carry=CIN  dbl_ovrd=off  block_type=constant
  carryin3 : xbsIndex_r4/Constant  arith_type=Unsigned  const=0  n_bits=1  bin_pt=0  explicit_period=on  period=1  equ=P=C  opselect=C  inp2=PCIN>>17  opr=+  inp1=P  carry=CIN  dbl_ovrd=off  block_type=constant
  carryinsel3 : xbsIndex_r4/Constant  arith_type=Unsigned  const=0  n_bits=3  bin_pt=0  explicit_period=on  period=1  equ=P=C  opselect=C  inp2=PCIN>>17  opr=+  inp1=P  carry=CIN  dbl_ovrd=off  block_type=constant
  negate_dsp48 : xbsIndex_r4/DSP48E  use_a=Direct from A Port  use_b=Direct from B Port  reset_preg=off  pattern_from_creg=off  pattern='000000000000'  mask_from_creg=off  pattern_mask='3FFFFFFFFFFF'  sel_rounding_mask=Select mask  use_op=off  use_creg=off  rst_all=off  en_all=off  use_pcin=off  use_carrycascin=off  use_multsignin=off  use_carryout=off  use_patterndetect=off  use_patternbdetect=off  use_overflow=off  use_underflow=off  use_acout=off  use_bcout=off  use_pcout=on  use_multsignout=off  use_carrycascout=off  pipeline_a=1  pipeline_b=1  pipeline_acout=1  pipeline_bcout=1  pipeline_c=on  pipeline_p=on  pipeline_mult=on  pipeline_opmode=on  pipeline_alumode=on  pipeline_carryin=on  pipeline_carryinsel=on  rst_a=off  rst_b=off  rst_c=off  rst_mult=off  rst_p=off  rst_carry_in=off  rst_alumode=off  rst_ctrl=off  en_a1=off  en_a2=off  en_b1=off  en_b2=off  en_c=off  en_mult=off  en_p=off  en_carry_in=off  en_alumode=off  en_multcarryin=off  en_ctrl=off  use_synth_model=off  addsub_mode=ONE48  xl_useadderonly=off  block_type=dsp48e
      settings: block_version=10.1.3
  opcode1 : xbsIndex_r4/Constant  arith_type=Signed (2's comp)  const=-1  n_bits=18  bin_pt=0  explicit_period=on  period=1  equ=P=C  opselect=C  inp2=PCIN>>17  opr=+  inp1=P  carry=CIN  dbl_ovrd=off  block_type=constant
  opcode3 : xbsIndex_r4/Constant  arith_type=Unsigned  const=5  n_bits=7  bin_pt=0  explicit_period=on  period=1  equ=P=C  opselect=C  inp2=PCIN>>17  opr=+  inp1=P  carry=CIN  dbl_ovrd=off  block_type=constant
  Out1 : Outport
  pcout : Outport  Port=2
  wires:
  Convert1/1 -> Out1/1
  Reinterpret/1 -> Convert1/1
  carryinsel3/1 -> negate_dsp48/6
  carryin3/1 -> negate_dsp48/5
  alucode3/1 -> negate_dsp48/4
  opcode3/1 -> negate_dsp48/3
  Convert/1 -> Reinterpret1/1
  In1/1 -> Convert/1
  negate_dsp48/1 -> Reinterpret/1
  negate_dsp48/2 -> pcout/1
  Reinterpret1/1 -> negate_dsp48/1
  opcode1/1 -> negate_dsp48/2

== system monroe_library/unscr_tail/complex_addsub1 ==
  a : Inport
  b : Inport  Port=2
  Convert{,1..3} (4 alike) : xbsIndex_r4/Convert  arith_type="Signed  (2's comp)"  n_bits=BitWidth  bin_pt=BitWidth - 1  quantization=Truncate  overflow=Wrap  en=off  latency=add_latency  dbl_ovrd=off  pipeline=off  block_type=convert
      settings: xl_area=[0, 0, 0, 0, 0, 0, 0]
  Shift{,1..3} (4 alike) : xbsIndex_r4/Shift  shift_dir=Right  shift_bits=1  en=off  latency=0  precision=Full  arith_type="Signed  (2's comp)"  n_bits=8  bin_pt=2  quantization=Truncate  overflow=Wrap  dbl_ovrd=off  block_type=shift
      settings: xl_area=[0, 0, 0, 0, 0, 0, 0]  block_version=9.1.01
  c_to_ri : casper_library/Misc/c_to_ri  SystemSampleTime=-1  n_bits=BitWidth  bin_pt=BitWidth-1
      settings: AttributesFormatString=18_17 r/i
  c_to_ri1 : casper_library/Misc/c_to_ri  SystemSampleTime=-1  n_bits=BitWidth  bin_pt=BitWidth-1
      settings: AttributesFormatString=18_17 r/i
  dsp48_complex_add : Subsystem  mask{a_bit_width=BitWidth, a_bin_pt=BitWidth-2, bw_bit_width=BitWidth, bw_bin_pt=BitWidth-2}
      mask prompts: a_bit_width "'a' bit width"; a_bin_pt "'a' binary point"; bw_bit_width "'bw' bit width"; bw_bin_pt "'bw' binary point"
  ri_to_c : casper_library/Misc/ri_to_c  SystemSampleTime=-1
  ri_to_c1 : casper_library/Misc/ri_to_c  SystemSampleTime=-1
  a+b : Outport
  a-b : Outport  Port=2
  wires:
  Convert3/1 -> ri_to_c1/1
  Convert1/1 -> ri_to_c1/2
  c_to_ri/1 -> dsp48_complex_add/3(bw_re)
  c_to_ri/2 -> dsp48_complex_add/2(a_im)
  c_to_ri1/1 -> dsp48_complex_add/1(a_re)
  c_to_ri1/2 -> dsp48_complex_add/4(bw_im)
  Convert/1 -> ri_to_c/1
  Convert2/1 -> ri_to_c/2
  a/1 -> c_to_ri/1
  ri_to_c/1 -> a+b/1
  ri_to_c1/1 -> a-b/1
  b/1 -> c_to_ri1/1
  Shift/1 -> Convert/1
  Shift1/1 -> Convert1/1
  Shift2/1 -> Convert2/1
  Shift3/1 -> Convert3/1
  dsp48_complex_add/3(a-bw_re) -> Shift1/1
  dsp48_complex_add/4(a-bw_im) -> Shift2/1
  dsp48_complex_add/2(a+bw_im) -> Shift3/1
  dsp48_complex_add/1(a+bw_re) -> Shift/1

== system monroe_library/unscr_tail/complex_addsub2 ==
  a : Inport
  b : Inport  Port=2
  Convert{,1..3} (4 alike) : xbsIndex_r4/Convert  arith_type="Signed  (2's comp)"  n_bits=BitWidth  bin_pt=BitWidth - 1  quantization=Truncate  overflow=Wrap  en=off  latency=add_latency  dbl_ovrd=off  pipeline=off  block_type=convert
      settings: xl_area=[0, 0, 0, 0, 0, 0, 0]
  Shift{,1..3} (4 alike) : xbsIndex_r4/Shift  shift_dir=Right  shift_bits=1  en=off  latency=0  precision=Full  arith_type="Signed  (2's comp)"  n_bits=8  bin_pt=2  quantization=Truncate  overflow=Wrap  dbl_ovrd=off  block_type=shift
      settings: xl_area=[0, 0, 0, 0, 0, 0, 0]  block_version=9.1.01
  c_to_ri : casper_library/Misc/c_to_ri  SystemSampleTime=-1  n_bits=BitWidth  bin_pt=BitWidth-1
      settings: AttributesFormatString=18_17 r/i
  c_to_ri1 : casper_library/Misc/c_to_ri  SystemSampleTime=-1  n_bits=BitWidth  bin_pt=BitWidth-1
      settings: AttributesFormatString=18_17 r/i
  dsp48_complex_add : Subsystem  mask{a_bit_width=BitWidth, a_bin_pt=BitWidth-2, bw_bit_width=BitWidth, bw_bin_pt=BitWidth-2}
      mask prompts: a_bit_width "'a' bit width"; a_bin_pt "'a' binary point"; bw_bit_width "'bw' bit width"; bw_bin_pt "'bw' binary point"
  ri_to_c : casper_library/Misc/ri_to_c  SystemSampleTime=-1
  ri_to_c1 : casper_library/Misc/ri_to_c  SystemSampleTime=-1
  a+b : Outport
  a-b : Outport  Port=2
  wires:
  dsp48_complex_add/1(a+bw_re) -> Shift/1
  dsp48_complex_add/2(a+bw_im) -> Shift3/1
  dsp48_complex_add/4(a-bw_im) -> Shift2/1
  dsp48_complex_add/3(a-bw_re) -> Shift1/1
  Shift3/1 -> Convert3/1
  Shift2/1 -> Convert2/1
  Shift1/1 -> Convert1/1
  Shift/1 -> Convert/1
  b/1 -> c_to_ri1/1
  ri_to_c1/1 -> a-b/1
  ri_to_c/1 -> a+b/1
  a/1 -> c_to_ri/1
  Convert2/1 -> ri_to_c/2
  Convert/1 -> ri_to_c/1
  c_to_ri1/2 -> dsp48_complex_add/4(bw_im)
  c_to_ri1/1 -> dsp48_complex_add/1(a_re)
  c_to_ri/2 -> dsp48_complex_add/2(a_im)
  c_to_ri/1 -> dsp48_complex_add/3(bw_re)
  Convert1/1 -> ri_to_c1/2
  Convert3/1 -> ri_to_c1/1

== system monroe_library/unscr_tail/mirror_spectrum ==
  sync : Inport
  din0 : Inport  Port=2
  reo_in0 : Inport  Port=3
  din1 : Inport  Port=4
  reo_in1 : Inport  Port=5
  din2 : Inport  Port=6
  reo_in2 : Inport  Port=7
  din3 : Inport  Port=8
  reo_in3 : Inport  Port=9
  Delay1 : xbsIndex_r4/Delay  en=off  latency=3  dbl_ovrd=off  reg_retiming=off  block_type=delay
  Delay2 : xbsIndex_r4/Delay  en=off  latency=1  dbl_ovrd=off  reg_retiming=off  block_type=delay
  Delay3 : S-Function  LoadFcn=xlBlockLoadCallback(gcbh);  FunctionName=sysgen  Parameters=ptable_  EnableBusSupport=off  mask(Xilinx Delay Block){infoedit=Hardware notes: A delay line is a chain, each link of which is an SRL16 followed by a flip-flop., en_sgadvanced=, en=off, latency=bram_latency + 1 + reorder_din_latency, dbl_ovrd_sgadvanced=, dbl_ovrd=off, reg_retiming_sgadvanced=, reg_retiming=off, xl_use_area_sgadvanced=, xl_use_area=off, xl_area=[0,0,0,0,0,0,0], has_advanced_control=0, sggui_pos=-1,-1,-1,-1, block_type=delay, block_version=, sg_icon_stat=60,56,1,1,white,blue,0,83e6bb61,right,,[ ],[ ], sg_mask_display=|, sg_list_contents=, sg_blockgui_xml=}
      mask sg_mask_display=|
      | fprintf('','COMMENT: begin icon graphics');
      | patch([0 60 60 0 0 ],[0 0 56 56 0 ],[0.77 0.82 0.91 ]);
      | plot([0 60 60 0 0 ],[0 0 56 56 0 ]);
      | patch([12.2 23.76 31.76 39.76 47.76 31.76 20.2 12.2 ],[36.88 36.88 44.88 36.88 44.88 44.88 44.88 36.88 ],[1 1 1 ]);
      | patch([20.2 31.76 23.76 12.2 20.2 ],[28.88 28.88 36.88 36.88 28.88 ],[0.931 0.946 0.973 ]);
      | patch([12.2 23.76 31.76 20.2 12.2 ],[20.88 20.88 28.88 28.88 20.88 ],[1 1 1 ]);
      | patch([20.2 47.76 39.76 31.76 23.76 12.2 20.2 ],[12.88 12.88 20.88 12.88 20.88 20.88 12.88 ],[0.931 0.946 0.973 ]);
      | fprintf('','COMMENT: end icon graphics');
      | fprintf('','COMMENT: begin icon text');
      |
      |
      | color('black');disp('z^{-3}','texmode','on');
      | fprintf('','COMMENT: end icon text');
      mask prompts: infoedit ""; en_sgadvanced ""; en "Provide enable port"; dbl_ovrd_sgadvanced ""; dbl_ovrd "Override with doubles"; reg_retiming_sgadvanced ""; reg_retiming "Implement using behavioral HDL."; xl_use_area_sgadvanced ""; xl_use_area "Define FPGA area for resource estimation"; xl_area "FPGA area [slices, FFs, BRAMs, LUTs, IOBs, emb. mults, TBUFs]"; has_advanced_control ""; sggui_pos ""; block_type ""; block_version ""; sg_icon_stat ""; sg_mask_display ""; sg_list_contents ""; sg_blockgui_xml ""
      mask help: Hardware notes: A delay line is a chain, each link of which is an SRL16 followed by a flip-flop.
      mask init: same as monroe_library/counter_limited_fast/Delay1
      settings: CopyFcn=xlBlockMoveCallback(gcbh);  DeleteFcn=xlDestroyGui(gcbh);  ModelCloseFcn=xlDestroyGui(gcbh);  PreSaveFcn=xlBlockPreSaveCallback(gcbh);  PostSaveFcn=xlBlockPostSaveCallback(gcbh);  DestroyFcn=xlDestroyGui(gcbh);  OpenFcn=xlOpenGui(gcbh, 'delay_gui.xml', @xlmagicenablement, -1)  CloseFcn=xlDestroyGui(gcbh);  MoveFcn=xlBlockMoveCallback(gcbh);
      mask Help: eval('');xlDoc('-book','sysgen','-topic','Delay');
      mask Display:
      | fprintf('','COMMENT: begin icon graphics');
      | patch([0 60 60 0 0 ],[0 0 56 56 0 ],[0.77 0.82 0.91 ]);
      | plot([0 60 60 0 0 ],[0 0 56 56 0 ]);
      | patch([12.2 23.76 31.76 39.76 47.76 31.76 20.2 12.2 ],[36.88 36.88 44.88 36.88 44.88 44.88 44.88 36.88 ],[1 1 1 ]);
      | patch([20.2 31.76 23.76 12.2 20.2 ],[28.88 28.88 36.88 36.88 28.88 ],[0.931 0.946 0.973 ]);
      | patch([12.2 23.76 31.76 20.2 12.2 ],[20.88 20.88 28.88 28.88 20.88 ],[1 1 1 ]);
      | patch([20.2 47.76 39.76 31.76 23.76 12.2 20.2 ],[12.88 12.88 20.88 12.88 20.88 20.88 12.88 ],[0.931 0.946 0.973 ]);
      | fprintf('','COMMENT: end icon graphics');
      | fprintf('','COMMENT: begin icon text');
      | 
      | 
      | color('black');disp('z^{-3}','texmode','on');
      | fprintf('','COMMENT: end icon text');
  Delay4 : S-Function  LoadFcn=xlBlockLoadCallback(gcbh);  FunctionName=sysgen  Parameters=ptable_  EnableBusSupport=off  mask(Xilinx Delay Block){infoedit=Hardware notes: A delay line is a chain, each link of which is an SRL16 followed by a flip-flop., en_sgadvanced=, en=off, latency=bram_latency + 1 + reorder_din_latency, dbl_ovrd_sgadvanced=, dbl_ovrd=off, reg_retiming_sgadvanced=, reg_retiming=off, xl_use_area_sgadvanced=, xl_use_area=off, xl_area=[0,0,0,0,0,0,0], has_advanced_control=0, sggui_pos=-1,-1,-1,-1, block_type=delay, block_version=, sg_icon_stat=60,56,1,1,white,blue,0,83e6bb61,right,,[ ],[ ], sg_mask_display=|, sg_list_contents=, sg_blockgui_xml=}
      mask sg_mask_display=|
      | fprintf('','COMMENT: begin icon graphics');
      | patch([0 60 60 0 0 ],[0 0 56 56 0 ],[0.77 0.82 0.91 ]);
      | plot([0 60 60 0 0 ],[0 0 56 56 0 ]);
      | patch([12.2 23.76 31.76 39.76 47.76 31.76 20.2 12.2 ],[36.88 36.88 44.88 36.88 44.88 44.88 44.88 36.88 ],[1 1 1 ]);
      | patch([20.2 31.76 23.76 12.2 20.2 ],[28.88 28.88 36.88 36.88 28.88 ],[0.931 0.946 0.973 ]);
      | patch([12.2 23.76 31.76 20.2 12.2 ],[20.88 20.88 28.88 28.88 20.88 ],[1 1 1 ]);
      | patch([20.2 47.76 39.76 31.76 23.76 12.2 20.2 ],[12.88 12.88 20.88 12.88 20.88 20.88 12.88 ],[0.931 0.946 0.973 ]);
      | fprintf('','COMMENT: end icon graphics');
      | fprintf('','COMMENT: begin icon text');
      |
      |
      | color('black');disp('z^{-3}','texmode','on');
      | fprintf('','COMMENT: end icon text');
      mask prompts: infoedit ""; en_sgadvanced ""; en "Provide enable port"; dbl_ovrd_sgadvanced ""; dbl_ovrd "Override with doubles"; reg_retiming_sgadvanced ""; reg_retiming "Implement using behavioral HDL."; xl_use_area_sgadvanced ""; xl_use_area "Define FPGA area for resource estimation"; xl_area "FPGA area [slices, FFs, BRAMs, LUTs, IOBs, emb. mults, TBUFs]"; has_advanced_control ""; sggui_pos ""; block_type ""; block_version ""; sg_icon_stat ""; sg_mask_display ""; sg_list_contents ""; sg_blockgui_xml ""
      mask help: Hardware notes: A delay line is a chain, each link of which is an SRL16 followed by a flip-flop.
      mask init: same as monroe_library/counter_limited_fast/Delay1
      settings: CopyFcn=xlBlockMoveCallback(gcbh);  DeleteFcn=xlDestroyGui(gcbh);  ModelCloseFcn=xlDestroyGui(gcbh);  PreSaveFcn=xlBlockPreSaveCallback(gcbh);  PostSaveFcn=xlBlockPostSaveCallback(gcbh);  DestroyFcn=xlDestroyGui(gcbh);  OpenFcn=xlOpenGui(gcbh, 'delay_gui.xml', @xlmagicenablement, -1)  CloseFcn=xlDestroyGui(gcbh);  MoveFcn=xlBlockMoveCallback(gcbh);
      mask Help: eval('');xlDoc('-book','sysgen','-topic','Delay');
      mask Display:
      | fprintf('','COMMENT: begin icon graphics');
      | patch([0 60 60 0 0 ],[0 0 56 56 0 ],[0.77 0.82 0.91 ]);
      | plot([0 60 60 0 0 ],[0 0 56 56 0 ]);
      | patch([12.2 23.76 31.76 39.76 47.76 31.76 20.2 12.2 ],[36.88 36.88 44.88 36.88 44.88 44.88 44.88 36.88 ],[1 1 1 ]);
      | patch([20.2 31.76 23.76 12.2 20.2 ],[28.88 28.88 36.88 36.88 28.88 ],[0.931 0.946 0.973 ]);
      | patch([12.2 23.76 31.76 20.2 12.2 ],[20.88 20.88 28.88 28.88 20.88 ],[1 1 1 ]);
      | patch([20.2 47.76 39.76 31.76 23.76 12.2 20.2 ],[12.88 12.88 20.88 12.88 20.88 20.88 12.88 ],[0.931 0.946 0.973 ]);
      | fprintf('','COMMENT: end icon graphics');
      | fprintf('','COMMENT: begin icon text');
      | 
      | 
      | color('black');disp('z^{-3}','texmode','on');
      | fprintf('','COMMENT: end icon text');
  Delay5 : xbsIndex_r4/Delay  en=off  latency=bram_latency + 1 + reorder_din_latency  dbl_ovrd=off  reg_retiming=off  block_type=delay
  Delay6 : S-Function  LoadFcn=xlBlockLoadCallback(gcbh);  FunctionName=sysgen  Parameters=ptable_  EnableBusSupport=off  mask(Xilinx Delay Block){infoedit=Hardware notes: A delay line is a chain, each link of which is an SRL16 followed by a flip-flop., en_sgadvanced=, en=off, latency=bram_latency + 1 + reorder_din_latency, dbl_ovrd_sgadvanced=, dbl_ovrd=off, reg_retiming_sgadvanced=, reg_retiming=off, xl_use_area_sgadvanced=, xl_use_area=off, xl_area=[0,0,0,0,0,0,0], has_advanced_control=0, sggui_pos=-1,-1,-1,-1, block_type=delay, block_version=, sg_icon_stat=60,56,1,1,white,blue,0,83e6bb61,right,,[ ],[ ], sg_mask_display=|, sg_list_contents=, sg_blockgui_xml=}
      mask sg_mask_display=|
      | fprintf('','COMMENT: begin icon graphics');
      | patch([0 60 60 0 0 ],[0 0 56 56 0 ],[0.77 0.82 0.91 ]);
      | plot([0 60 60 0 0 ],[0 0 56 56 0 ]);
      | patch([12.2 23.76 31.76 39.76 47.76 31.76 20.2 12.2 ],[36.88 36.88 44.88 36.88 44.88 44.88 44.88 36.88 ],[1 1 1 ]);
      | patch([20.2 31.76 23.76 12.2 20.2 ],[28.88 28.88 36.88 36.88 28.88 ],[0.931 0.946 0.973 ]);
      | patch([12.2 23.76 31.76 20.2 12.2 ],[20.88 20.88 28.88 28.88 20.88 ],[1 1 1 ]);
      | patch([20.2 47.76 39.76 31.76 23.76 12.2 20.2 ],[12.88 12.88 20.88 12.88 20.88 20.88 12.88 ],[0.931 0.946 0.973 ]);
      | fprintf('','COMMENT: end icon graphics');
      | fprintf('','COMMENT: begin icon text');
      |
      |
      | color('black');disp('z^{-3}','texmode','on');
      | fprintf('','COMMENT: end icon text');
      mask prompts: infoedit ""; en_sgadvanced ""; en "Provide enable port"; dbl_ovrd_sgadvanced ""; dbl_ovrd "Override with doubles"; reg_retiming_sgadvanced ""; reg_retiming "Implement using behavioral HDL."; xl_use_area_sgadvanced ""; xl_use_area "Define FPGA area for resource estimation"; xl_area "FPGA area [slices, FFs, BRAMs, LUTs, IOBs, emb. mults, TBUFs]"; has_advanced_control ""; sggui_pos ""; block_type ""; block_version ""; sg_icon_stat ""; sg_mask_display ""; sg_list_contents ""; sg_blockgui_xml ""
      mask help: Hardware notes: A delay line is a chain, each link of which is an SRL16 followed by a flip-flop.
      mask init: same as monroe_library/counter_limited_fast/Delay1
      settings: CopyFcn=xlBlockMoveCallback(gcbh);  DeleteFcn=xlDestroyGui(gcbh);  ModelCloseFcn=xlDestroyGui(gcbh);  PreSaveFcn=xlBlockPreSaveCallback(gcbh);  PostSaveFcn=xlBlockPostSaveCallback(gcbh);  DestroyFcn=xlDestroyGui(gcbh);  OpenFcn=xlOpenGui(gcbh, 'delay_gui.xml', @xlmagicenablement, -1)  CloseFcn=xlDestroyGui(gcbh);  MoveFcn=xlBlockMoveCallback(gcbh);
      mask Help: eval('');xlDoc('-book','sysgen','-topic','Delay');
      mask Display:
      | fprintf('','COMMENT: begin icon graphics');
      | patch([0 60 60 0 0 ],[0 0 56 56 0 ],[0.77 0.82 0.91 ]);
      | plot([0 60 60 0 0 ],[0 0 56 56 0 ]);
      | patch([12.2 23.76 31.76 39.76 47.76 31.76 20.2 12.2 ],[36.88 36.88 44.88 36.88 44.88 44.88 44.88 36.88 ],[1 1 1 ]);
      | patch([20.2 31.76 23.76 12.2 20.2 ],[28.88 28.88 36.88 36.88 28.88 ],[0.931 0.946 0.973 ]);
      | patch([12.2 23.76 31.76 20.2 12.2 ],[20.88 20.88 28.88 28.88 20.88 ],[1 1 1 ]);
      | patch([20.2 47.76 39.76 31.76 23.76 12.2 20.2 ],[12.88 12.88 20.88 12.88 20.88 20.88 12.88 ],[0.931 0.946 0.973 ]);
      | fprintf('','COMMENT: end icon graphics');
      | fprintf('','COMMENT: begin icon text');
      | 
      | 
      | color('black');disp('z^{-3}','texmode','on');
      | fprintf('','COMMENT: end icon text');
  Subsystem : Subsystem
  Subsystem1 : Subsystem
  Subsystem2 : Subsystem
  Subsystem3 : Subsystem
  cram1 : Subsystem
  cram2 : Subsystem
  cram3 : Subsystem
  cram4 : Subsystem
  delay_uncram_{0..3} (4 alike) : xbsIndex_r4/Delay  en=off  latency=2  dbl_ovrd=off  reg_retiming=off  block_type=delay
  dsp48_negate_dual : monroe_library/dsp48_negate_dual  SystemSampleTime=-1  a_bit_width=input_bit_width  a_bin_pt=input_bit_width-1
  dsp48_negate_dual1 : monroe_library/dsp48_negate_dual  SystemSampleTime=-1  a_bit_width=input_bit_width  a_bin_pt=input_bit_width-1
  sel_gen : Subsystem
  uncram1 : Subsystem
  uncram2 : Subsystem
  uncram3 : Subsystem
  uncram4 : Subsystem
  sync_out : Outport
  dout0 : Outport  Port=2
  dout1 : Outport  Port=3
  dout2 : Outport  Port=4
  dout3 : Outport  Port=5
  wires:
  sel_gen/1(sel_out) -> Subsystem/1(In1), Subsystem3/1(In1), Subsystem2/1(In1), Subsystem1/1(In1)
  Delay1/1 -> sel_gen/1(sync_in), Delay2/1
  cram4/1(out) -> Subsystem3/3(In4)
  dsp48_negate_dual1/2 -> cram4/2(in1)
  delay_uncram_3/1 -> cram4/1(in0)
  cram3/1(out) -> Subsystem2/3(In4)
  dsp48_negate_dual1/1 -> cram3/2(in1)
  delay_uncram_2/1 -> cram3/1(in0)
  cram2/1(out) -> Subsystem1/3(In4)
  dsp48_negate_dual/2 -> cram2/2(in1)
  delay_uncram_1/1 -> cram2/1(in0)
  cram1/1(out) -> Subsystem/3(In4)
  dsp48_negate_dual/1 -> cram1/2(in1)
  delay_uncram_0/1 -> cram1/1(in0)
  uncram4/2(out1) -> dsp48_negate_dual1/2
  uncram3/2(out1) -> dsp48_negate_dual1/1
  uncram2/2(out1) -> dsp48_negate_dual/2
  uncram1/2(out1) -> dsp48_negate_dual/1
  Subsystem3/1(Out1) -> dout3/1
  Delay6/1 -> Subsystem3/2(In3)
  Subsystem2/1(Out1) -> dout2/1
  Delay4/1 -> Subsystem2/2(In3)
  Subsystem1/1(Out1) -> dout1/1
  Delay3/1 -> Subsystem1/2(In3)
  Delay5/1 -> Subsystem/2(In3)
  din3/1 -> Delay6/1
  din0/1 -> Delay5/1
  din1/1 -> Delay3/1
  din2/1 -> Delay4/1
  Delay2/1 -> sync_out/1
  sync/1 -> Delay1/1
  uncram4/1(out0) -> delay_uncram_3/1
  uncram3/1(out0) -> delay_uncram_2/1
  uncram2/1(out0) -> delay_uncram_1/1
  uncram1/1(out0) -> delay_uncram_0/1
  reo_in3/1 -> uncram4/1(in)
  reo_in2/1 -> uncram3/1(in)
  reo_in1/1 -> uncram2/1(in)
  reo_in0/1 -> uncram1/1(in)
  Subsystem/1(Out1) -> dout0/1
